simulink library "mconversion16Lib"  (Simulink 7.1)
settings Model: Creator=awarlock  LastModifiedBy=zren  ExtModeAutoUpdateStatusClock=off

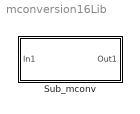
== system mconversion16Lib ==
  Sub_mconv : Subsystem  TreatAsAtomicUnit=on

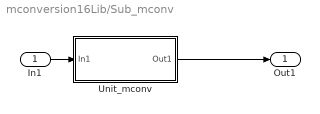
== system mconversion16Lib/Sub_mconv ==
  In1 : Inport  OutDataType=sfix(16)  OutScaling=2^0
  Unit_mconv : Subsystem  TreatAsAtomicUnit=on
  Out1 : Outport  OutDataType=sfix(16)  OutScaling=2^0
  wires:
  In1/1 -> Unit_mconv/1(In1)
  Unit_mconv/1(Out1) -> Out1/1

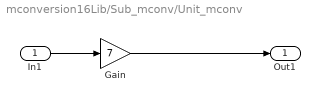
== system mconversion16Lib/Sub_mconv/Unit_mconv ==
  In1 : Inport  OutDataType=sfix(16)  OutScaling=2^0
  Gain : Gain  Gain=7  ParameterDataType=sfix(16)  ParameterScaling=2^0  OutDataType=sfix(16)  OutScaling=2^0
  Out1 : Outport  OutDataType=sfix(16)  OutScaling=2^0
  wires:
  In1/1 -> Gain/1
  Gain/1 -> Out1/1
